simulink model "quadcopter"  (R2024a)
settings: Solver=ode45  StartTime=0.0  StopTime=100  FixedStep=0.0001  RelTol=1e-3
libraries: slpidlib x9
(part 2 of 2)

== matlab function quadcopter/Guidance/Processer ==
  settings: updateMethod=DISCRETE  sampleTime=0.05
  data: pos input; X_cmd output; Y_cmd output; Z_cmd output; path_matrix input size=[200, 3]
function [X_cmd, Y_cmd, Z_cmd] = fcn(pos, path_matrix)
    persistent current_wp_idx num_wp
    
    if isempty(current_wp_idx)
        current_wp_idx = 2; 
        num_wp = size(path_matrix, 1);
    end
    
    pos = pos(:);
    lookahead_distance = 2.0; 
    
    if current_wp_idx > num_wp
        target = path_matrix(end, :)';
    else
        A = path_matrix(current_wp_idx - 1, :)';
        B = path_matrix(current_wp_idx, :)';
        
        path_vec = B - A;
        path_length = norm(path_vec);
        
        if path_length < 0.001
            u = [0;0;0]; 
        else
            u = path_vec / path_length;
        end
        
        drone_vec = pos - A;
        along_path_dist = dot(drone_vec, u);
        rabbit_dist = along_path_dist + lookahead_distance;
        
        if rabbit_dist >= path_length
            current_wp_idx = current_wp_idx + 1;
            target = B; 
        else
            target = A + rabbit_dist * u;
        end
    end
    
    % Raw outputs, strictly managed by external Simulink blocks now
    X_cmd = target(1); Y_cmd = target(2); Z_cmd = target(3);
end

== matlab function quadcopter/Visualization/PositionErrorVisualization ==
  settings: updateMethod=DISCRETE  sampleTime=0.005
  data: pos_cmd input; pos_act input; position_error output
function position_error = fcn(pos_cmd, pos_act)
    e_x = pos_cmd(1) - pos_act(1);
    e_y = pos_cmd(2) - pos_act(2);
    e_z = pos_cmd(3) - pos_act(3);

    position_error = sqrt(e_x^2 + e_y^2 + e_z^2);
end
